simulink model "wheel_dynamics"  (R2023b)
settings: Solver=VariableStepAuto  StartTime=0.0  StopTime=10.0  RelTol=1e-3
undefined symbols (not defined in the file or in its folder): tire_loaded_radius
settings Model: Creator=bglen  LastModifiedBy=bglen

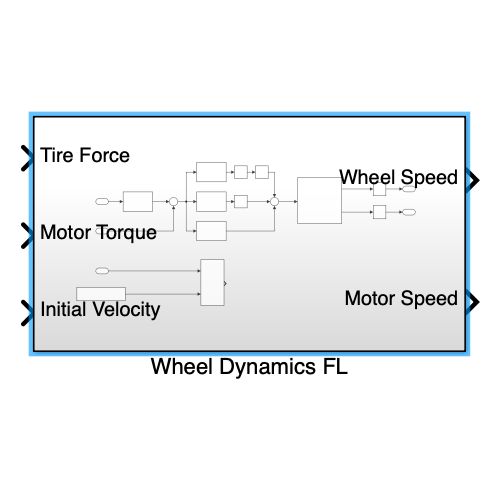
[thumbnail: Simulink's stored preview of the top-level diagram]
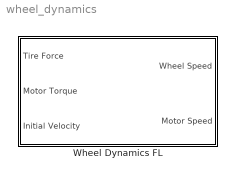
== system wheel_dynamics ==
  Wheel Dynamics FL : Subsystem

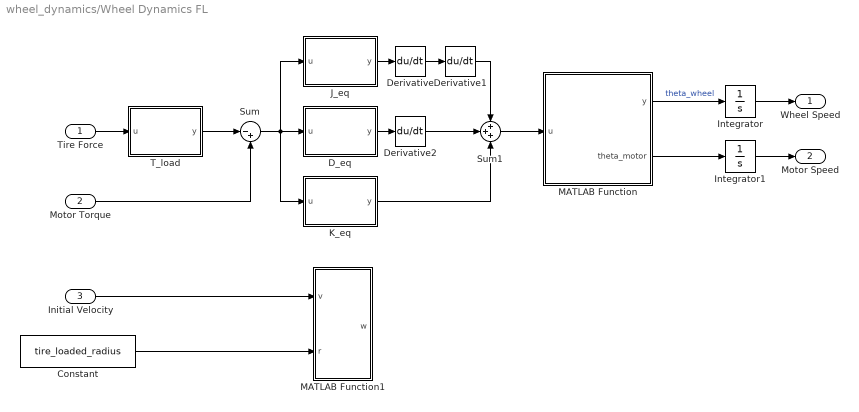
== system wheel_dynamics/Wheel Dynamics FL ==
  Tire Force : Inport
  Motor Torque : Inport  Port=2
  Initial Velocity : Inport  Port=3
  Constant : Constant  Value=tire_loaded_radius
  D_eq : MATLAB Function  TreatAsAtomicUnit=on
  Derivative : Derivative
  Derivative1 : Derivative
  Derivative2 : Derivative
  Integrator : Integrator
  Integrator1 : Integrator
  J_eq : MATLAB Function  TreatAsAtomicUnit=on
  K_eq : MATLAB Function  TreatAsAtomicUnit=on
  MATLAB Function : MATLAB Function  TreatAsAtomicUnit=on
  MATLAB Function1 : MATLAB Function  TreatAsAtomicUnit=on
  Sum : Sum  Inputs=|-+
  Sum1 : Sum  Inputs=+++
  T_load : MATLAB Function  TreatAsAtomicUnit=on
  Wheel Speed : Outport
  Motor Speed : Outport  Port=2
  wires:
  Motor Torque/1 -> Sum/2
  Tire Force/1 -> T_load/1(u)
  T_load/1(y) -> Sum/1
  Integrator/1 -> Wheel Speed/1
  Sum/1 -> D_eq/1(u), K_eq/1(u), J_eq/1(u)
  J_eq/1(y) -> Derivative/1
  Derivative/1 -> Derivative1/1
  D_eq/1(y) -> Derivative2/1
  Derivative2/1 -> Sum1/2
  Derivative1/1 -> Sum1/1
  K_eq/1(y) -> Sum1/3
  Sum1/1 -> MATLAB Function/1(u)
  MATLAB Function/1(y) -> Integrator/1  "theta_wheel"
  MATLAB Function/2(theta_motor) -> Integrator1/1
  Integrator1/1 -> Motor Speed/1
  Initial Velocity/1 -> MATLAB Function1/1(v)
  Constant/1 -> MATLAB Function1/2(r)

== matlab function wheel_dynamics/Wheel Dynamics FL/T_load ==
  data: u input; y output
function y = fcn(u)

r=1; % wheel radius
N1=1; % gear ratio
N2=1; % gear ratio

T_load=r*N1/N2*u; % 'load torque' calculation

y = u;

== matlab function wheel_dynamics/Wheel Dynamics FL/D_eq ==
  data: u input; y output
function y = fcn(u)

% frictions
D1=0; % gear 1
D2=0; % gear 2
Dm=0; % motor
Dw=0; % wheel

Da=D1+Dm;
Db=D2+Dw;

N1=1; % gear ratio
N2=1; % gear ratio

Deq=Da+Db*(N1/N2)^2; % equivalent friction

y = Deq*u;

== matlab function wheel_dynamics/Wheel Dynamics FL/K_eq ==
  data: u input; y output
function y = fcn(u)

% spring / stiffness
Ks2=0; % shaft 2
Ks1=0; % shaft 1

Ka=Ks1;
Kb=Ks2;

N1=1; % gear ratio
N2=1; % gear ratio

Keq=Ka+Kb*(N1/N2)^2; % equivalent spring / stiffness

y = Keq*u;

== matlab function wheel_dynamics/Wheel Dynamics FL/MATLAB Function ==
  data: u input; y output; theta_motor output
function [y, theta_motor]= fcn(u)

N1=1; % gear ratio
N2=1; % gear ratio

theta_motor=1/u;
theta_wheel=theta_motor*N2/N1;

y = theta_wheel;

== matlab function wheel_dynamics/Wheel Dynamics FL/MATLAB Function1 ==
  data: v input; w output; r input
function w = fcn(v, r)

w = v/r;

== matlab function wheel_dynamics/Wheel Dynamics FL/J_eq ==
  data: u input; y output
function y = fcn(u)

% inertias
J1=1; % gear 1
J2=1; % gear 2
Js2=1; % shaft 2
Js1=1; % shaft 1
Jm=1; % motor
Jw=1; % wheel

Ja=J1+Js1+Jm;
Jb=J2+Js2+Jw;

N1=1; % gear ratio
N2=1; % gear ratio

Jeq=Ja+Jb*(N1/N2)^2; % equivalent inertia

y = Jeq*u;
